simulink model "Scratch2_Mota"  (R2016a)
settings: Solver=ode5  SolverMode=SingleTasking  StartTime=0.0  StopTime=Ttot  FixedStep=min(Ts_phy,Ts_sim)  RelTol=1e-3
PreLoadFcn:
  | Electrical_model_settings_Scratch2_Mota
InitFcn:
  | Electrical_model_settings_Scratch2_Mota
values from neighbouring files (symbols this model uses):
  col = {}    [oog_example_init.m]
  flex = {}    [oog_example_init.m]
  systemBase = {}    [oog_example_init.m]
  Ts = Ts_c    (= 0.0001)    [oog_example_init.m]
  Ts_phy = 1*Ts_sim    (= 0.0001)    [oog_example_init.m]
  Ts_sim = 100e-6    (= 0.0001)    [oog_example_init.m]
  wt1 = {}    [oog_example_init.m]
  wt2 = wt1    [oog_example_init.m]
  wt3 = wt1    [oog_example_init.m]
undefined symbols (not defined in the file or in its folder): avr, D1, Delta, DiscIntNeverNeededParam, governor, interface, Lf1, sm
libraries: powerlib x49, simulink_extras x35, pwrsysBasic x30, powerlib_meascontrol x17, pwrsysVICtrl x15, simulink x5, pwrsysVSrc x4, pwrsysTransf x4
(part 3 of 3)

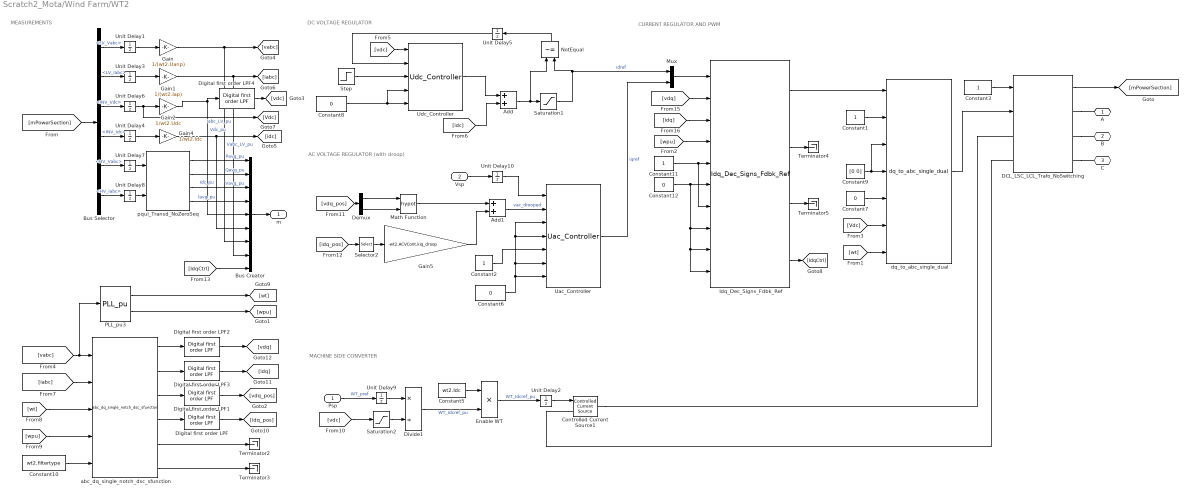
== system Scratch2_Mota/Wind Farm/WT2 ==
  note: MEASUREMENTS
  note: MACHINE SIDE CONVERTER
  note: AC VOLTAGE REGULATOR (with droop)
  note: DC VOLTAGE REGULATOR
  note: CURRENT REGULATOR AND PWM
  Psp : Inport
  Vsp : Inport  Port=2
  Add : Sum
  Add1 : Sum
  Bus Creator : BusCreator  Inputs=9
  Bus Selector : BusSelector  OutputSignals=LV_Vabc,LV_Iabc,INV_Vdc,INV_Idc,HV_Vabc,HV_Iabc
  Constant{1..3,11} (4 alike) : Constant  SampleTime=wt2.Ts_control
  Constant10 : Constant  Value=wt2.filtertype  SampleTime=wt2.Ts_control
  Constant{6..8,12} (4 alike) : Constant  Value=0  SampleTime=wt2.Ts_control
  Constant5 : Constant  Value=wt2.Idc  SampleTime=wt2.Ts_control
  Constant9 : Constant  Value=[0 0]  SampleTime=wt2.Ts_control
  Controlled Current Source1 : powerlib/Electrical Sources/Controlled Current Source  Initialize=on  Source_Type=DC  Amplitude=0  Phase=0  Frequency=50  Measurements=None
  DCL_LSC_LCL_Trafo_NoSwitching : pwrsysVSrc/DCL_LSC_LCL_Trafo_NoSwitching  Sn=wt2.Sn  fn=systemBase.fn  Uhv_ab=col.Un  Uab=wt2.Un  lf2=wt2.LCL.l2  rf2=wt2.LCL.r2  Lf1=wt2.LCL.L1  Rf1=wt2.LCL.R1  Cf=wt2.LCL.Cf  Rc=wt2.LCL.Rf  Cdc=wt2.Cdc  Udc0=wt2.Udc  Tsm=wt2.Ts_control  Tstart=wt2.DCVCont.Start
  Demux : Demux  Outputs=2
  Digital first order LPF{,1..4} (5 alike) : pwrsysBasic/Digital first order LPF  Ts=wt2.Ts_control  fcutout=wt2.CurrCont.f_LPF_noise
  Divide1 : Product  Inputs=*/
  Enable WT : Product  Inputs=**
  Gain : Gain  Gain=1/(wt2.Uanp)
  Gain1 : Gain  Gain=1/(wt2.Iap)
  Gain2 : Gain  Gain=1/wt2.Udc
  Gain4 : Gain  Gain=1/wt2.Idc
  Gain5 : Gain  Gain=-wt2.ACVCont.kiq_droop
  Idq_Dec_Signs_Fdbk_Ref : pwrsysVICtrl/Idq_Dec_Signs_Fdbk_Ref  Ts=wt2.Ts_control  fn=systemBase.fn  Kp=wt2.CurrContSingle.kp  Ti=wt2.CurrContSingle.Ti  L=wt2.CurrCont.x  PI_max=wt2.CurrCont.PImax  PI_min=wt2.CurrCont.PImin  TrafoPhaseComp=0
  Math Function : Math  Operator=hypot  SaturateOnIntegerOverflow=on
  Mux : Mux  Inputs=2
  NotEqual : RelationalOperator  Operator=~=  OutDataTypeStr=boolean
  PLL_pu3 : pwrsysBasic/PLL_pu  fn=systemBase.fn  Ts=wt2.Ts_control  Kp_pll=90  Ki_pll=1200  Kd_pll=0  PLL_ini=60
  Saturation1 : Saturate  UpperLimit=wt2.DCVCont.PImax  LowerLimit=wt2.DCVCont.PImin
  Saturation2 : Saturate  UpperLimit=1.2  LowerLimit=0.8
  Selector2 : Selector  IndexMode=Zero-based  InputPortWidth=2  IndexOptions=Index vector (dialog)  Indices=1  OutputSizes=1
  Step : Step  Time=wt2.DCVCont.Start  SampleTime=0
  Terminator{2..5} (4 alike) : Terminator
  Uac_Controller : pwrsysVICtrl/Uac_Controller  Ts=wt2.Ts_control  Kg=wt2.ACVCont.kg  Kp=wt2.ACVCont.kp  Ti=wt2.ACVCont.Ti  PI_max=wt2.ACVCont.PImax  PI_min=wt2.ACVCont.PImin
  Udc_Controller : pwrsysVICtrl/Udc_Controller  Ts=wt2.Ts_control  Kp=wt2.DCVContSingle.kp  Ti=wt2.DCVContSingle.Ti  PI_max=wt2.DCVCont.PImax  PI_min=wt2.DCVCont.PImin
  Unit Delay{1,3,7..8} (4 alike) : UnitDelay  InitialCondition=[0 0 0]  SampleTime=wt2.Ts_control
  Unit Delay10 : UnitDelay  InitialCondition=1  SampleTime=wt2.Ts_control
  Unit Delay{2,4..5,9} (4 alike) : UnitDelay  SampleTime=wt2.Ts_control
  Unit Delay6 : UnitDelay  InitialCondition=1  SampleTime=wt2.Ts_control
  abc_dq_single_notch_dsc_sfunction : pwrsysTransf/abc_dq_single_notch_dsc_sfunction  Ts=wt2.Ts_control  fn=2*systemBase.fn  zeta=wt2.CurrCont.zeta
  dq_to_abc_single_dual : pwrsysVICtrl/dq_to_abc_single_dual  Ts=wt2.Ts_control  Uabp=wt2.Uabp
  pqui_Transd_NoZeroSeq : pwrsysBasic/pqui_Transd_NoZeroSeq  Sn=wt2.Sn  Uanp=col.Uanp  Iap=wt2.Iap*(wt2.Un/col.Un)
  A : PMIOPort  Port=1  Side=Right
  B : PMIOPort  Port=2  Side=Right
  C : PMIOPort  Port=3  Side=Right
  m : Outport
  wires:
  Divide1/1 -> Enable WT/2  "WT_Idcref_pu"
  Bus Selector/1 -> Unit Delay1/1  "<LV_Vabc>"
  [idq_pos] -> Selector2/1
  Unit Delay2/1 -> Controlled Current Source1/1
  Gain1/1 -> Bus Creator/8, [iabc]  "Iabc_LV_pu"
  Bus Selector/2 -> Unit Delay3/1  "<LV_Iabc>"
  Gain5/1 -> Add1/2
  Math Function/1 -> Add1/1
  Constant6/1 -> Uac_Controller/7, Uac_Controller/6, Uac_Controller/3, Uac_Controller/4
  Constant5/1 -> Enable WT/1
  Add1/1 -> Uac_Controller/2  "vac_drooped"
  Vsp/1 -> Unit Delay10/1
  [mPowerSection] -> Bus Selector/1
  Enable WT/1 -> Unit Delay2/1  "WT_Idcref_pu"
  Gain/1 -> Bus Creator/7, [vabc]  "Vabc_LV_pu"
  Constant2/1 -> Uac_Controller/5
  Constant8/1 -> Udc_Controller/4, Udc_Controller/5
  NotEqual/1 -> Unit Delay5/1
  [vdc] -> Udc_Controller/1
  Unit Delay5/1 -> Udc_Controller/2
  Saturation1/1 -> NotEqual/2, Mux/1  "idref"
  [idc] -> Add/2
  Udc_Controller/1 -> Add/1
  Add/1 -> NotEqual/1, Saturation1/1
  Step/1 -> Udc_Controller/3
  [idq] -> Idq_Dec_Signs_Fdbk_Ref/3
  [Vdc] -> dq_to_abc_single_dual/6
  [wpu] -> Idq_Dec_Signs_Fdbk_Ref/4
  dq_to_abc_single_dual/1 -> DCL_LSC_LCL_Trafo_NoSwitching/2
  Mux/1 -> Idq_Dec_Signs_Fdbk_Ref/1
  Constant3/1 -> DCL_LSC_LCL_Trafo_NoSwitching/1
  Saturation2/1 -> Divide1/2
  Psp/1 -> Unit Delay9/1  "WT_pref"
  [vdc] -> Saturation2/1
  [wt] -> dq_to_abc_single_dual/7
  Constant10/1 -> abc_dq_single_notch_dsc_sfunction/5
  Bus Selector/5 -> Unit Delay7/1  "<HV_Vabc>"
  Bus Selector/6 -> Unit Delay8/1  "<HV_Iabc>"
  pqui_Transd_NoZeroSeq/1 -> Bus Creator/1  "Pavg_pu"
  pqui_Transd_NoZeroSeq/2 -> Bus Creator/2  "Qavg_pu"
  pqui_Transd_NoZeroSeq/3 -> Bus Creator/3  "Vavg_pu"
  pqui_Transd_NoZeroSeq/4 -> Bus Creator/4  "Iavg_pu"
  Bus Creator/1 -> m/1
  Bus Selector/3 -> Unit Delay6/1  "<INV_Vdc>"
  Gain2/1 -> Bus Creator/5, Digital first order LPF4/1  "Vdc_pu"
  Gain4/1 -> [idc], Bus Creator/6  "Idc_pu"
  Bus Selector/4 -> Unit Delay4/1  "<INV_Idc>"
  PLL_pu3/2 -> [wpu]
  PLL_pu3/1 -> [wt]
  Uac_Controller/1 -> Mux/2  "iqref"
  DCL_LSC_LCL_Trafo_NoSwitching/1 -> [mPowerSection]
  Unit Delay1/1 -> Gain/1
  Unit Delay3/1 -> Gain1/1
  Unit Delay4/1 -> Gain4/1
  Unit Delay8/1 -> pqui_Transd_NoZeroSeq/2
  Unit Delay6/1 -> [Vdc], Gain2/1
  Unit Delay7/1 -> pqui_Transd_NoZeroSeq/1
  Unit Delay9/1 -> Divide1/1
  Unit Delay10/1 -> Uac_Controller/1
  abc_dq_single_notch_dsc_sfunction/6 -> Terminator3/1
  abc_dq_single_notch_dsc_sfunction/5 -> Terminator2/1
  Selector2/1 -> Gain5/1
  Idq_Dec_Signs_Fdbk_Ref/2 -> Terminator4/1
  [vdq] -> Idq_Dec_Signs_Fdbk_Ref/2
  Constant1/1 -> dq_to_abc_single_dual/2
  Constant7/1 -> dq_to_abc_single_dual/5
  Constant9/1 -> dq_to_abc_single_dual/4, dq_to_abc_single_dual/3
  Constant11/1 -> Idq_Dec_Signs_Fdbk_Ref/7, Idq_Dec_Signs_Fdbk_Ref/5
  Constant12/1 -> Idq_Dec_Signs_Fdbk_Ref/8, Idq_Dec_Signs_Fdbk_Ref/9, Idq_Dec_Signs_Fdbk_Ref/10, Idq_Dec_Signs_Fdbk_Ref/6
  Idq_Dec_Signs_Fdbk_Ref/3 -> Terminator5/1
  Idq_Dec_Signs_Fdbk_Ref/4 -> [IdqCtrl]
  [IdqCtrl] -> Bus Creator/9
  Idq_Dec_Signs_Fdbk_Ref/1 -> dq_to_abc_single_dual/1
  [wt] -> abc_dq_single_notch_dsc_sfunction/3
  [wpu] -> abc_dq_single_notch_dsc_sfunction/4
  abc_dq_single_notch_dsc_sfunction/1 -> Digital first order LPF2/1
  [vabc] -> abc_dq_single_notch_dsc_sfunction/1, PLL_pu3/1
  [iabc] -> abc_dq_single_notch_dsc_sfunction/2
  abc_dq_single_notch_dsc_sfunction/3 -> Digital first order LPF1/1
  abc_dq_single_notch_dsc_sfunction/4 -> Digital first order LPF/1
  abc_dq_single_notch_dsc_sfunction/2 -> Digital first order LPF3/1
  Digital first order LPF/1 -> [idq_pos]
  Digital first order LPF1/1 -> [vdq_pos]
  [vdq_pos] -> Demux/1
  Demux/1 -> Math Function/1
  Demux/2 -> Math Function/2
  Digital first order LPF2/1 -> [vdq]
  Digital first order LPF3/1 -> [idq]
  Digital first order LPF4/1 -> [vdc]
  connections:
  Controlled Current Source1/RConn1 -- DCL_LSC_LCL_Trafo_NoSwitching/LConn1
  DCL_LSC_LCL_Trafo_NoSwitching/RConn3 -- C/RConn1
  DCL_LSC_LCL_Trafo_NoSwitching/RConn1 -- A/RConn1
  DCL_LSC_LCL_Trafo_NoSwitching/RConn2 -- B/RConn1
  Controlled Current Source1/LConn1 -- DCL_LSC_LCL_Trafo_NoSwitching/LConn2

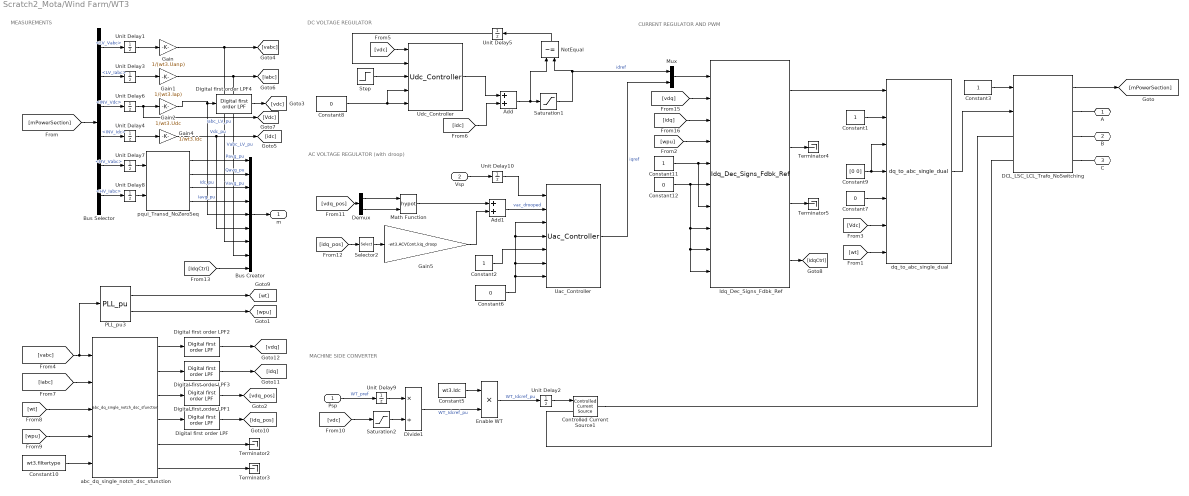
== system Scratch2_Mota/Wind Farm/WT3 ==
  note: MEASUREMENTS
  note: MACHINE SIDE CONVERTER
  note: AC VOLTAGE REGULATOR (with droop)
  note: DC VOLTAGE REGULATOR
  note: CURRENT REGULATOR AND PWM
  Psp : Inport
  Vsp : Inport  Port=2
  Add : Sum
  Add1 : Sum
  Bus Creator : BusCreator  Inputs=9
  Bus Selector : BusSelector  OutputSignals=LV_Vabc,LV_Iabc,INV_Vdc,INV_Idc,HV_Vabc,HV_Iabc
  Constant{1..3,11} (4 alike) : Constant  SampleTime=wt3.Ts_control
  Constant10 : Constant  Value=wt3.filtertype  SampleTime=wt3.Ts_control
  Constant{6..8,12} (4 alike) : Constant  Value=0  SampleTime=wt3.Ts_control
  Constant5 : Constant  Value=wt3.Idc  SampleTime=wt3.Ts_control
  Constant9 : Constant  Value=[0 0]  SampleTime=wt3.Ts_control
  Controlled Current Source1 : powerlib/Electrical Sources/Controlled Current Source  Initialize=on  Source_Type=DC  Amplitude=0  Phase=0  Frequency=50  Measurements=None
  DCL_LSC_LCL_Trafo_NoSwitching : pwrsysVSrc/DCL_LSC_LCL_Trafo_NoSwitching  Sn=wt3.Sn  fn=systemBase.fn  Uhv_ab=col.Un  Uab=wt3.Un  lf2=wt3.LCL.l2  rf2=wt3.LCL.r2  Lf1=wt3.LCL.L1  Rf1=wt3.LCL.R1  Cf=wt3.LCL.Cf  Rc=wt3.LCL.Rf  Cdc=wt3.Cdc  Udc0=wt3.Udc  Tsm=wt3.Ts_control  Tstart=wt3.DCVCont.Start
  Demux : Demux  Outputs=2
  Digital first order LPF{,1..4} (5 alike) : pwrsysBasic/Digital first order LPF  Ts=wt3.Ts_control  fcutout=wt3.CurrCont.f_LPF_noise
  Divide1 : Product  Inputs=*/
  Enable WT : Product  Inputs=**
  Gain : Gain  Gain=1/(wt3.Uanp)
  Gain1 : Gain  Gain=1/(wt3.Iap)
  Gain2 : Gain  Gain=1/wt3.Udc
  Gain4 : Gain  Gain=1/wt3.Idc
  Gain5 : Gain  Gain=-wt3.ACVCont.kiq_droop
  Idq_Dec_Signs_Fdbk_Ref : pwrsysVICtrl/Idq_Dec_Signs_Fdbk_Ref  Ts=wt3.Ts_control  fn=systemBase.fn  Kp=wt3.CurrContSingle.kp  Ti=wt3.CurrContSingle.Ti  L=wt3.CurrCont.x  PI_max=wt3.CurrCont.PImax  PI_min=wt3.CurrCont.PImin  TrafoPhaseComp=0
  Math Function : Math  Operator=hypot  SaturateOnIntegerOverflow=on
  Mux : Mux  Inputs=2
  NotEqual : RelationalOperator  Operator=~=  OutDataTypeStr=boolean
  PLL_pu3 : pwrsysBasic/PLL_pu  fn=systemBase.fn  Ts=wt3.Ts_control  Kp_pll=90  Ki_pll=1200  Kd_pll=0  PLL_ini=60
  Saturation1 : Saturate  UpperLimit=wt3.DCVCont.PImax  LowerLimit=wt3.DCVCont.PImin
  Saturation2 : Saturate  UpperLimit=1.2  LowerLimit=0.8
  Selector2 : Selector  IndexMode=Zero-based  InputPortWidth=2  IndexOptions=Index vector (dialog)  Indices=1  OutputSizes=1
  Step : Step  Time=wt3.DCVCont.Start  SampleTime=0
  Terminator{2..5} (4 alike) : Terminator
  Uac_Controller : pwrsysVICtrl/Uac_Controller  Ts=wt3.Ts_control  Kg=wt3.ACVCont.kg  Kp=wt3.ACVCont.kp  Ti=wt3.ACVCont.Ti  PI_max=wt3.ACVCont.PImax  PI_min=wt3.ACVCont.PImin
  Udc_Controller : pwrsysVICtrl/Udc_Controller  Ts=wt3.Ts_control  Kp=wt3.DCVContSingle.kp  Ti=wt3.DCVContSingle.Ti  PI_max=wt3.DCVCont.PImax  PI_min=wt3.DCVCont.PImin
  Unit Delay{1,3,7..8} (4 alike) : UnitDelay  InitialCondition=[0 0 0]  SampleTime=wt3.Ts_control
  Unit Delay10 : UnitDelay  InitialCondition=1  SampleTime=wt3.Ts_control
  Unit Delay{2,4..5,9} (4 alike) : UnitDelay  SampleTime=wt3.Ts_control
  Unit Delay6 : UnitDelay  InitialCondition=1  SampleTime=wt3.Ts_control
  abc_dq_single_notch_dsc_sfunction : pwrsysTransf/abc_dq_single_notch_dsc_sfunction  Ts=wt3.Ts_control  fn=2*systemBase.fn  zeta=wt3.CurrCont.zeta
  dq_to_abc_single_dual : pwrsysVICtrl/dq_to_abc_single_dual  Ts=wt3.Ts_control  Uabp=wt3.Uabp
  pqui_Transd_NoZeroSeq : pwrsysBasic/pqui_Transd_NoZeroSeq  Sn=wt3.Sn  Uanp=col.Uanp  Iap=wt3.Iap*(wt3.Un/col.Un)
  A : PMIOPort  Port=1  Side=Right
  B : PMIOPort  Port=2  Side=Right
  C : PMIOPort  Port=3  Side=Right
  m : Outport
  wires:
  Divide1/1 -> Enable WT/2  "WT_Idcref_pu"
  Bus Selector/1 -> Unit Delay1/1  "<LV_Vabc>"
  [idq_pos] -> Selector2/1
  Unit Delay2/1 -> Controlled Current Source1/1
  Gain1/1 -> Bus Creator/8, [iabc]  "Iabc_LV_pu"
  Bus Selector/2 -> Unit Delay3/1  "<LV_Iabc>"
  Gain5/1 -> Add1/2
  Math Function/1 -> Add1/1
  Constant6/1 -> Uac_Controller/7, Uac_Controller/6, Uac_Controller/3, Uac_Controller/4
  Constant5/1 -> Enable WT/1
  Add1/1 -> Uac_Controller/2  "vac_drooped"
  Vsp/1 -> Unit Delay10/1
  [mPowerSection] -> Bus Selector/1
  Enable WT/1 -> Unit Delay2/1  "WT_Idcref_pu"
  Gain/1 -> Bus Creator/7, [vabc]  "Vabc_LV_pu"
  Constant2/1 -> Uac_Controller/5
  Constant8/1 -> Udc_Controller/4, Udc_Controller/5
  NotEqual/1 -> Unit Delay5/1
  [vdc] -> Udc_Controller/1
  Unit Delay5/1 -> Udc_Controller/2
  Saturation1/1 -> NotEqual/2, Mux/1  "idref"
  [idc] -> Add/2
  Udc_Controller/1 -> Add/1
  Add/1 -> NotEqual/1, Saturation1/1
  Step/1 -> Udc_Controller/3
  [idq] -> Idq_Dec_Signs_Fdbk_Ref/3
  [Vdc] -> dq_to_abc_single_dual/6
  [wpu] -> Idq_Dec_Signs_Fdbk_Ref/4
  dq_to_abc_single_dual/1 -> DCL_LSC_LCL_Trafo_NoSwitching/2
  Mux/1 -> Idq_Dec_Signs_Fdbk_Ref/1
  Constant3/1 -> DCL_LSC_LCL_Trafo_NoSwitching/1
  Saturation2/1 -> Divide1/2
  Psp/1 -> Unit Delay9/1  "WT_pref"
  [vdc] -> Saturation2/1
  [wt] -> dq_to_abc_single_dual/7
  Constant10/1 -> abc_dq_single_notch_dsc_sfunction/5
  Bus Selector/5 -> Unit Delay7/1  "<HV_Vabc>"
  Bus Selector/6 -> Unit Delay8/1  "<HV_Iabc>"
  pqui_Transd_NoZeroSeq/1 -> Bus Creator/1  "Pavg_pu"
  pqui_Transd_NoZeroSeq/2 -> Bus Creator/2  "Qavg_pu"
  pqui_Transd_NoZeroSeq/3 -> Bus Creator/3  "Vavg_pu"
  pqui_Transd_NoZeroSeq/4 -> Bus Creator/4  "Iavg_pu"
  Bus Creator/1 -> m/1
  Bus Selector/3 -> Unit Delay6/1  "<INV_Vdc>"
  Gain2/1 -> Digital first order LPF4/1, Bus Creator/5  "Vdc_pu"
  Gain4/1 -> [idc], Bus Creator/6  "Idc_pu"
  Bus Selector/4 -> Unit Delay4/1  "<INV_Idc>"
  PLL_pu3/2 -> [wpu]
  PLL_pu3/1 -> [wt]
  Uac_Controller/1 -> Mux/2  "iqref"
  DCL_LSC_LCL_Trafo_NoSwitching/1 -> [mPowerSection]
  Unit Delay1/1 -> Gain/1
  Unit Delay3/1 -> Gain1/1
  Unit Delay4/1 -> Gain4/1
  Unit Delay8/1 -> pqui_Transd_NoZeroSeq/2
  Unit Delay6/1 -> [Vdc], Gain2/1
  Unit Delay7/1 -> pqui_Transd_NoZeroSeq/1
  Unit Delay9/1 -> Divide1/1
  Unit Delay10/1 -> Uac_Controller/1
  abc_dq_single_notch_dsc_sfunction/6 -> Terminator3/1
  abc_dq_single_notch_dsc_sfunction/5 -> Terminator2/1
  Selector2/1 -> Gain5/1
  Idq_Dec_Signs_Fdbk_Ref/2 -> Terminator4/1
  [vdq] -> Idq_Dec_Signs_Fdbk_Ref/2
  Constant1/1 -> dq_to_abc_single_dual/2
  Constant7/1 -> dq_to_abc_single_dual/5
  Constant9/1 -> dq_to_abc_single_dual/4, dq_to_abc_single_dual/3
  Constant11/1 -> Idq_Dec_Signs_Fdbk_Ref/7, Idq_Dec_Signs_Fdbk_Ref/5
  Constant12/1 -> Idq_Dec_Signs_Fdbk_Ref/8, Idq_Dec_Signs_Fdbk_Ref/9, Idq_Dec_Signs_Fdbk_Ref/10, Idq_Dec_Signs_Fdbk_Ref/6
  Idq_Dec_Signs_Fdbk_Ref/3 -> Terminator5/1
  Idq_Dec_Signs_Fdbk_Ref/4 -> [IdqCtrl]
  [IdqCtrl] -> Bus Creator/9
  Idq_Dec_Signs_Fdbk_Ref/1 -> dq_to_abc_single_dual/1
  [wt] -> abc_dq_single_notch_dsc_sfunction/3
  [wpu] -> abc_dq_single_notch_dsc_sfunction/4
  abc_dq_single_notch_dsc_sfunction/1 -> Digital first order LPF2/1
  [vabc] -> abc_dq_single_notch_dsc_sfunction/1, PLL_pu3/1
  [iabc] -> abc_dq_single_notch_dsc_sfunction/2
  abc_dq_single_notch_dsc_sfunction/3 -> Digital first order LPF1/1
  abc_dq_single_notch_dsc_sfunction/4 -> Digital first order LPF/1
  abc_dq_single_notch_dsc_sfunction/2 -> Digital first order LPF3/1
  Digital first order LPF/1 -> [idq_pos]
  Digital first order LPF1/1 -> [vdq_pos]
  [vdq_pos] -> Demux/1
  Demux/1 -> Math Function/1
  Demux/2 -> Math Function/2
  Digital first order LPF2/1 -> [vdq]
  Digital first order LPF3/1 -> [idq]
  Digital first order LPF4/1 -> [vdc]
  connections:
  Controlled Current Source1/RConn1 -- DCL_LSC_LCL_Trafo_NoSwitching/LConn1
  DCL_LSC_LCL_Trafo_NoSwitching/RConn3 -- C/RConn1
  DCL_LSC_LCL_Trafo_NoSwitching/RConn1 -- A/RConn1
  DCL_LSC_LCL_Trafo_NoSwitching/RConn2 -- B/RConn1
  Controlled Current Source1/LConn1 -- DCL_LSC_LCL_Trafo_NoSwitching/LConn2

== system Scratch2_Mota/rms and power calc/LP filter 1 ==
  in : Inport
  Discrete Transfer Fcn (with initial outputs) : simulink_extras/Additional Discrete/Discrete Transfer Fcn (with initial outputs)  N=[1/tau*Ts/2 1/tau*Ts/2]  D=[(1/tau*Ts/2+1) (1/tau*Ts/2-1)]  U0=x0  Y0=y0  TS=Ts
  out : Outport
  wires:
  Discrete Transfer Fcn (with initial outputs)/1 -> out/1
  in/1 -> Discrete Transfer Fcn (with initial outputs)/1

== system Scratch2_Mota/rms and power calc/LP filter 66 ==
  in : Inport
  Discrete Transfer Fcn (with initial outputs) : simulink_extras/Additional Discrete/Discrete Transfer Fcn (with initial outputs)  N=[1/tau*Ts/2 1/tau*Ts/2]  D=[(1/tau*Ts/2+1) (1/tau*Ts/2-1)]  U0=x0  Y0=y0  TS=Ts
  out : Outport
  wires:
  Discrete Transfer Fcn (with initial outputs)/1 -> out/1
  in/1 -> Discrete Transfer Fcn (with initial outputs)/1

== system Scratch2_Mota/rms and power calc/Low pass filter P1 ==
  in : Inport
  Discrete Transfer Fcn (with initial outputs) : simulink_extras/Additional Discrete/Discrete Transfer Fcn (with initial outputs)  N=[1/tau*Ts/2 1/tau*Ts/2]  D=[(1/tau*Ts/2+1) (1/tau*Ts/2-1)]  U0=x0  Y0=y0  TS=Ts
  out : Outport
  wires:
  Discrete Transfer Fcn (with initial outputs)/1 -> out/1
  in/1 -> Discrete Transfer Fcn (with initial outputs)/1

== system Scratch2_Mota/rms and power calc/Low pass filter P2 ==
  in : Inport
  Discrete Transfer Fcn (with initial outputs) : simulink_extras/Additional Discrete/Discrete Transfer Fcn (with initial outputs)  N=[1/tau*Ts/2 1/tau*Ts/2]  D=[(1/tau*Ts/2+1) (1/tau*Ts/2-1)]  U0=x0  Y0=y0  TS=Ts
  out : Outport
  wires:
  Discrete Transfer Fcn (with initial outputs)/1 -> out/1
  in/1 -> Discrete Transfer Fcn (with initial outputs)/1

== system Scratch2_Mota/rms and power calc/Low pass filter P3 ==
  in : Inport
  Discrete Transfer Fcn (with initial outputs) : simulink_extras/Additional Discrete/Discrete Transfer Fcn (with initial outputs)  N=[1/tau*Ts/2 1/tau*Ts/2]  D=[(1/tau*Ts/2+1) (1/tau*Ts/2-1)]  U0=x0  Y0=y0  TS=Ts
  out : Outport
  wires:
  in/1 -> Discrete Transfer Fcn (with initial outputs)/1
  Discrete Transfer Fcn (with initial outputs)/1 -> out/1

== system Scratch2_Mota/rms and power calc/Low pass filter P4 ==
  in : Inport
  Discrete Transfer Fcn (with initial outputs) : simulink_extras/Additional Discrete/Discrete Transfer Fcn (with initial outputs)  N=[1/tau*Ts/2 1/tau*Ts/2]  D=[(1/tau*Ts/2+1) (1/tau*Ts/2-1)]  U0=x0  Y0=y0  TS=Ts
  out : Outport
  wires:
  in/1 -> Discrete Transfer Fcn (with initial outputs)/1
  Discrete Transfer Fcn (with initial outputs)/1 -> out/1

== system Scratch2_Mota/rms and power calc/Low pass filter Q ==
  in : Inport
  Discrete Transfer Fcn (with initial outputs) : simulink_extras/Additional Discrete/Discrete Transfer Fcn (with initial outputs)  N=[1/tau*Ts/2 1/tau*Ts/2]  D=[(1/tau*Ts/2+1) (1/tau*Ts/2-1)]  U0=x0  Y0=y0  TS=Ts
  out : Outport
  wires:
  Discrete Transfer Fcn (with initial outputs)/1 -> out/1
  in/1 -> Discrete Transfer Fcn (with initial outputs)/1

== system Scratch2_Mota/rms and power calc/Low pass filter Q1 ==
  in : Inport
  Discrete Transfer Fcn (with initial outputs) : simulink_extras/Additional Discrete/Discrete Transfer Fcn (with initial outputs)  N=[1/tau*Ts/2 1/tau*Ts/2]  D=[(1/tau*Ts/2+1) (1/tau*Ts/2-1)]  U0=x0  Y0=y0  TS=Ts
  out : Outport
  wires:
  Discrete Transfer Fcn (with initial outputs)/1 -> out/1
  in/1 -> Discrete Transfer Fcn (with initial outputs)/1

== system Scratch2_Mota/rms and power calc/Low pass filter Q2 ==
  in : Inport
  Discrete Transfer Fcn (with initial outputs) : simulink_extras/Additional Discrete/Discrete Transfer Fcn (with initial outputs)  N=[1/tau*Ts/2 1/tau*Ts/2]  D=[(1/tau*Ts/2+1) (1/tau*Ts/2-1)]  U0=x0  Y0=y0  TS=Ts
  out : Outport
  wires:
  in/1 -> Discrete Transfer Fcn (with initial outputs)/1
  Discrete Transfer Fcn (with initial outputs)/1 -> out/1

== system Scratch2_Mota/rms and power calc/Low pass filter Q3 ==
  in : Inport
  Discrete Transfer Fcn (with initial outputs) : simulink_extras/Additional Discrete/Discrete Transfer Fcn (with initial outputs)  N=[1/tau*Ts/2 1/tau*Ts/2]  D=[(1/tau*Ts/2+1) (1/tau*Ts/2-1)]  U0=x0  Y0=y0  TS=Ts
  out : Outport
  wires:
  in/1 -> Discrete Transfer Fcn (with initial outputs)/1
  Discrete Transfer Fcn (with initial outputs)/1 -> out/1

== system Scratch2_Mota/Automatic voltage regulator/PID_Governor1/LP filter power ==
  in : Inport
  Discrete Transfer Fcn (with initial outputs) : simulink_extras/Additional Discrete/Discrete Transfer Fcn (with initial outputs)  N=[1/tau*Ts/2 1/tau*Ts/2]  D=[(1/tau*Ts/2+1) (1/tau*Ts/2-1)]  U0=x0  Y0=y0  TS=Ts
  out : Outport
  wires:
  Discrete Transfer Fcn (with initial outputs)/1 -> out/1
  in/1 -> Discrete Transfer Fcn (with initial outputs)/1

== system Scratch2_Mota/SM_simple/powerCalcAndFilt1/LP filter frequency1 ==
  in : Inport
  Discrete Transfer Fcn (with initial outputs) : simulink_extras/Additional Discrete/Discrete Transfer Fcn (with initial outputs)  N=[1/tau*Ts/2 1/tau*Ts/2]  D=[(1/tau*Ts/2+1) (1/tau*Ts/2-1)]  U0=x0  Y0=y0  TS=Ts
  out : Outport
  wires:
  Discrete Transfer Fcn (with initial outputs)/1 -> out/1
  in/1 -> Discrete Transfer Fcn (with initial outputs)/1

== system Scratch2_Mota/SM_simple/powerCalcAndFilt1/LP filter frequency2 ==
  in : Inport
  Discrete Transfer Fcn (with initial outputs) : simulink_extras/Additional Discrete/Discrete Transfer Fcn (with initial outputs)  N=[1/tau*Ts/2 1/tau*Ts/2]  D=[(1/tau*Ts/2+1) (1/tau*Ts/2-1)]  U0=x0  Y0=y0  TS=Ts
  out : Outport
  wires:
  Discrete Transfer Fcn (with initial outputs)/1 -> out/1
  in/1 -> Discrete Transfer Fcn (with initial outputs)/1

== system Scratch2_Mota/Turbine Governor1/PID_Governor1/LP filter power ==
  in : Inport
  Discrete Transfer Fcn (with initial outputs) : simulink_extras/Additional Discrete/Discrete Transfer Fcn (with initial outputs)  N=[1/tau*Ts/2 1/tau*Ts/2]  D=[(1/tau*Ts/2+1) (1/tau*Ts/2-1)]  U0=x0  Y0=y0  TS=Ts
  out : Outport
  wires:
  Discrete Transfer Fcn (with initial outputs)/1 -> out/1
  in/1 -> Discrete Transfer Fcn (with initial outputs)/1
